simulink model "F16_mod"  (R2025b)
settings: Solver=ode4  StartTime=0  StopTime=Tend  FixedStep=0.01  RelTol=1e-3
values from neighbouring files (symbols this model uses):
  Param = load_F16_params()    [runF16_mod.m]
libraries: aerolibasang x3, aerolibobsolete x1, aerolibatmos2 x1
settings Model: Creator=sherpa  LastModifiedBy=karth
settings SolverCC: AlgebraicLoopSolver=TrustRegion
settings DataIOCC: SaveFormat=StructureWithTime
settings OptimizationCC: BlockReduction=off  DefaultParameterBehavior=Inlined  OptimizeBlockIOStorage=off  BufferReuse=off
settings DebuggingCC: AlgebraicLoopMsg=none  InitInArrayFormatMsg=none
settings ModelReferenceCC: EnableRefExpFcnMdlSchedulingChecks=on
settings RTWCC: GPUComputeCapability=3.5  DLArmComputeVersion=19.05

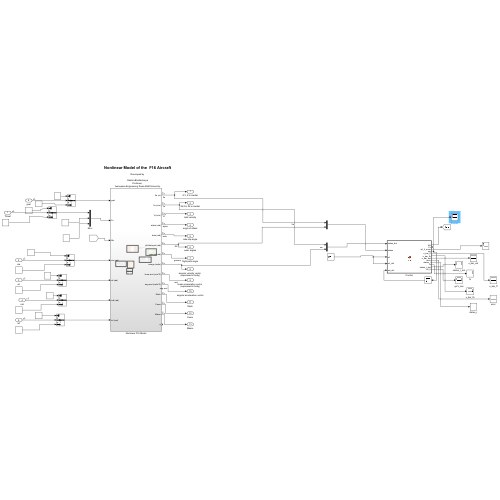
[thumbnail: Simulink's stored preview of the top-level diagram]
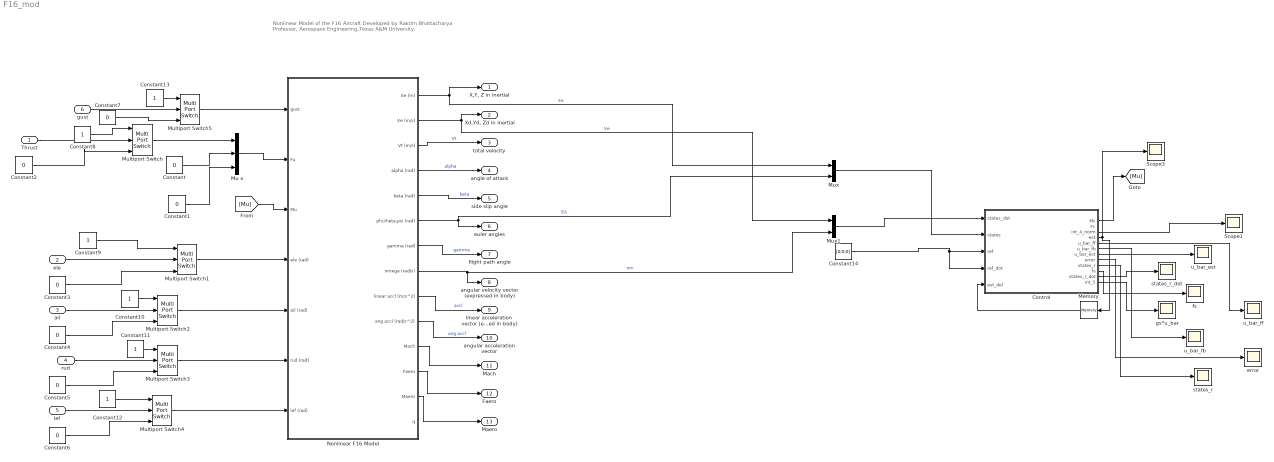
== system F16_mod ==
  note: Nonlinear Model of the F16 Aircraft
      |
      | Developed by
      |
      | Raktim Bhattacharya
      | Professor,
      | Aerospace Engineering,Texas A&M University.
  Thrust : Inport
  ele : Inport  Port=2
  ail : Inport  Port=3
  rud : Inport  Port=4
  lef : Inport  Port=5
  gust : Inport  Port=6
  Constant{,1..7} (8 alike) : Constant  Value=0
  Constant{8..13} (6 alike) : Constant
  Constant14 : Constant  Value=[0;0;0]
  Control : MATLAB Function  TreatAsAtomicUnit=on
  Memory : Memory  InitialCondition=[0;0;0]
  Mu x : Mux  Inputs=3
  Multiport Switch{,1..5} (6 alike) : MultiPortSwitch  DataPortOrder=Zero-based contiguous  Inputs=2  zeroidx=on  SaturateOnIntegerOverflow=off  InputSameDT=off
  Mux : Mux  Inputs=2
  Mux1 : Mux  Inputs=2
  Nonlinear F16 Model : Subsystem
  Scope1 : Scope
      settings: ActiveDisplayYMinimum=13407.32687  ActiveDisplayYMaximum=33407.32687  DataLoggingVariableName=ScopeData2
  Scope3 : Scope
      settings: ActiveDisplayYMinimum=-3.16857685066509  ActiveDisplayYMaximum=1.4182994151934736  DataLoggingVariableName=ScopeData4
  error : Scope
      settings: ActiveDisplayYMinimum=0.18819294431344591  ActiveDisplayYMaximum=1.6067438567419092  DataLoggingVariableName=ScopeData12
  fs : Scope
      settings: ActiveDisplayYMinimum=-3452.81147  ActiveDisplayYMaximum=2103.10858
  gs*u_bar : Scope
      settings: ActiveDisplayYMinimum=-2111.44761  ActiveDisplayYMaximum=3449.32295  DataLoggingVariableName=ScopeData2
  states_r : Scope
      settings: ActiveDisplayYMinimum=-1.0198079164284359  ActiveDisplayYMaximum=0.34149624108670595  DataLoggingVariableName=ScopeData3
  states_r_dot : Scope
      settings: ActiveDisplayYMinimum=-0.14936  ActiveDisplayYMaximum=0.22608  DataLoggingVariableName=ScopeData3
  u_bar_est : Scope
      settings: ActiveDisplayYMinimum=-0.14209  ActiveDisplayYMaximum=0.06478
  u_bar_fb : Scope
      settings: ActiveDisplayYMinimum=-1  ActiveDisplayYMaximum=1  DataLoggingVariableName=ScopeData11
  u_bar_ff : Scope
      settings: ActiveDisplayYMinimum=-3.90345245215E+6  ActiveDisplayYMaximum=3.513107206932E+7  DataLoggingVariableName=ScopeData15
  "X,Y, Z in inertial" : Outport
  "Xd,Yd, Zd in inertial" : Outport  Port=2
  total velocity : Outport  Port=3
  angle of attack : Outport  Port=4
  side slip angle : Outport  Port=5
  euler angles : Outport  Port=6
  flight path angle : Outport  Port=7
  angular velocity vector (expressed in body) : Outport  Port=8
  linear acceleration vector (expressed in body) : Outport  Port=9
  angular acceleration vector : Outport  Port=10
  Mach : Outport  Port=11
  Faero : Outport  Port=12
  Maero : Outport  Port=13
  wires:
  Nonlinear F16 Model/1(Xe (m)) -> "X,Y, Z in inertial"/1, Mux/1  "Xe"
  Nonlinear F16 Model/3(Vt (m/s)) -> total velocity/1  "Vt"
  Nonlinear F16 Model/4(alpha (rad)) -> angle of attack/1  "alpha"
  Nonlinear F16 Model/5(beta (rad)) -> side slip angle/1  "beta"
  Nonlinear F16 Model/7(gamma (rad)) -> flight path angle/1  "gamma"
  Nonlinear F16 Model/8(omega (rad/s)) -> angular velocity vector (expressed in body)/1, Mux1/2  "om"
  Nonlinear F16 Model/9(linear accl (m/s^2)) -> linear acceleration vector (expressed in body)/1  "accl"
  Nonlinear F16 Model/6(phi,theta,psi (rad)) -> euler angles/1, Mux/2  "EA"
  Nonlinear F16 Model/2(Ve (m/s)) -> "Xd,Yd, Zd in inertial"/1, Mux1/1  "Ve"
  Nonlinear F16 Model/10(ang accl (rad/s^2)) -> angular acceleration vector/1  "ang accl"
  Nonlinear F16 Model/11(Mach) -> Mach/1
  Nonlinear F16 Model/12(Faero) -> Faero/1
  Nonlinear F16 Model/13(Maero) -> Maero/1
  Control/1(Mc) -> [Mu]
  Control/5(u_bar_ff) -> u_bar_ff/1
  Control/9(states_r) -> states_r/1
  Control/6(u_bar_fb) -> u_bar_fb/1
  Control/3(int_4_norm) -> Scope1/1
  Memory/1 -> Control/5(est_del)
  Control/8(error) -> error/1
  Control/4(est) -> Memory/1, Scope3/1
  [Mu] -> Nonlinear F16 Model/3(Mu)
  Mux1/1 -> Control/1(states_dot)
  Constant/1 -> Mu x/2
  Mu x/1 -> Nonlinear F16 Model/2(Fu)
  Constant1/1 -> Mu x/3
  Thrust/1 -> Multiport Switch/2
  Multiport Switch/1 -> Mu x/1
  ele/1 -> Multiport Switch1/2
  Multiport Switch1/1 -> Nonlinear F16 Model/4(ele (rad))
  ail/1 -> Multiport Switch2/2
  Multiport Switch2/1 -> Nonlinear F16 Model/5(ail (rad))
  rud/1 -> Multiport Switch3/2
  Multiport Switch3/1 -> Nonlinear F16 Model/6(rud (rad))
  lef/1 -> Multiport Switch4/2
  Multiport Switch4/1 -> Nonlinear F16 Model/7(lef (rad))
  Constant2/1 -> Multiport Switch/3
  Constant3/1 -> Multiport Switch1/3
  Constant4/1 -> Multiport Switch2/3
  Constant5/1 -> Multiport Switch3/3
  Constant6/1 -> Multiport Switch4/3
  gust/1 -> Multiport Switch5/2
  Multiport Switch5/1 -> Nonlinear F16 Model/1(gust)
  Constant7/1 -> Multiport Switch5/3
  Constant8/1 -> Multiport Switch/1
  Constant9/1 -> Multiport Switch1/1
  Constant10/1 -> Multiport Switch2/1
  Constant11/1 -> Multiport Switch3/1
  Constant12/1 -> Multiport Switch4/1
  Constant13/1 -> Multiport Switch5/1
  Mux/1 -> Control/2(states)
  Constant14/1 -> Control/4(ref_dot), Control/3(ref)
  Control/7(u_bar_est) -> u_bar_est/1
  Control/10(fs) -> fs/1
  Control/12(int_5) -> gs*u_bar/1
  Control/11(states_r_dot) -> states_r_dot/1

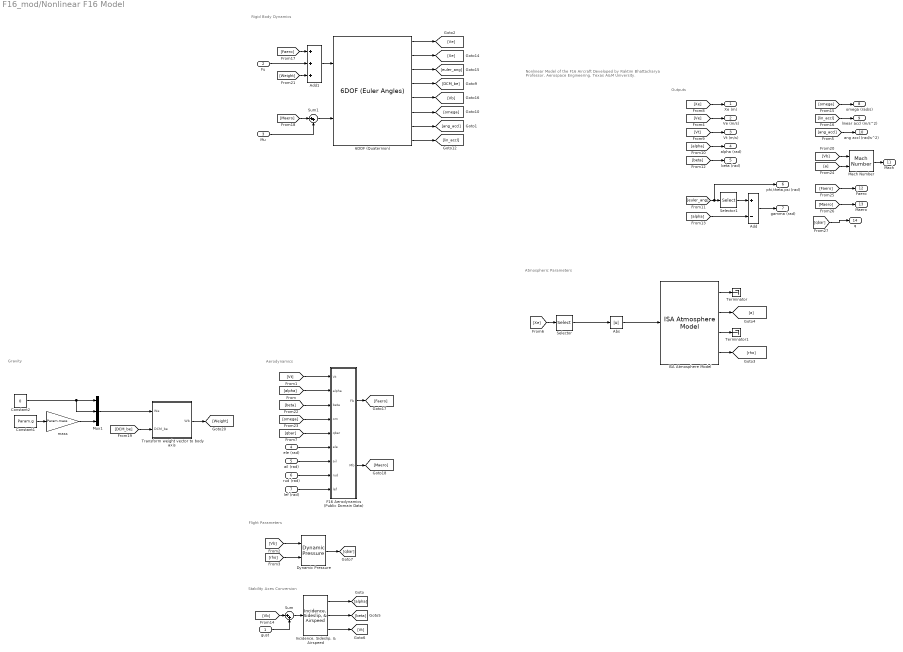
== system F16_mod/Nonlinear F16 Model ==
  note: Gravity
  note: Nonlinear Model of the F16 Aircraft
      |
      | Developed by Raktim Bhattacharya
      | Professor, Aerospace Engineering,
      | Texas A&M University.
  note: Aerodynamics
  note: Outputs
  note: Rigid Body Dynamics
  note: Stability Axes Conversion
  note: Atmospheric Parameters
  note: Flight Parameters
  gust : Inport  PortDimensions=3
  Fu : Inport  Port=2
  Mu : Inport  Port=3  PortDimensions=3
  ele (rad) : Inport  Port=4
  ail (rad) : Inport  Port=5
  rud (rad) : Inport  Port=6
  lef (rad) : Inport  Port=7
  6DOF (Quaternion) : aerolibobsolete/6DOF (Euler Angles)  units=Metric (MKS)  mtype=Fixed  rep=Euler Angles  xme_0=IC.inertial_position  Vm_0=IC.body_velocity  eul_0=IC.euler_angles  pm_0=IC.omega  mass_0=Param.mass  mass_e=0.5  mass_f=2.0  inertia=Param.moi  inertia_e=eye(3)  inertia_f=2*eye(3)  k_quat=1.0  vre_flag=on  abi_flag=off  aMode=0  xme_statename={'Xe', 'Ye', 'Ze'}  Vm_statename={'U', 'v', 'w'}  eul_statename=''  quat_statename={'qr', 'qi', 'qj', 'qk'}  pm_statename={'p', 'q', 'r'}  mass_statename=''
  Abs : Abs  SaturateOnIntegerOverflow=off
  Add : Sum  Inputs=+-
  Add1 : Sum  Inputs=+++
  Constant1 : Constant  Value=Param.g
  Constant2 : Constant  Value=0
  Dynamic Pressure : aerolibasang/Dynamic Pressure
  F16 Aerodynamics (Public Domain Data) : Subsystem
  ISA Atmosphere Model : aerolibatmos2/ISA Atmosphere Model  useExtended=off  action=Warning  custom=off  viscosityOut=off  g=9.80665  gamma=1.4  R=287.0531  L=0.0065  h_trop=11000  h_strat=20000  rho0=1.225  P0=101325  T0=288.15  h0=0  S=110.4  Tref=273.15  muref=1.716e-5
  "Incidence, Sideslip, & Airspeed" : aerolibasang/Incidence, Sideslip, & Airspeed
  Mach Number : aerolibasang/Mach Number
  Mux1 : Mux  Inputs=3
  Selector : Selector  InputPortWidth=3  IndexOptions=Index vector (dialog)  Indices=3  OutputSizes=1
  Selector1 : Selector  InputPortWidth=3  IndexOptions=Index vector (dialog)  Indices=2  OutputSizes=1
  Sum : Sum  Inputs=|++
  Sum1 : Sum  Inputs=|++
  Terminator : Terminator
  Terminator1 : Terminator
  Transform weight vector to body axis : MATLAB Function  TreatAsAtomicUnit=on
  mass : Gain  Gain=Param.mass
  Xe (m) : Outport
  Ve (m/s) : Outport  Port=2
  Vt (m/s) : Outport  Port=3
  alpha (rad) : Outport  Port=4
  beta (rad) : Outport  Port=5
  phi,theta,psi (rad) : Outport  Port=6
  gamma (rad) : Outport  Port=7
  omega (rad/s) : Outport  Port=8
  linear accl (m/s^2) : Outport  Port=9
  ang accl (rad/s^2) : Outport  Port=10
  Mach : Outport  Port=11
  Faero : Outport  Port=12
  Maero : Outport  Port=13
  q : Outport  Port=14
  wires:
  [Xe] -> Selector/1
  [beta] -> beta (rad)/1
  "Incidence, Sideslip, & Airspeed"/3 -> [Vt]
  ISA Atmosphere Model/3 -> Terminator1/1
  ISA Atmosphere Model/1 -> Terminator/1
  ISA Atmosphere Model/4 -> [rho]
  [rho] -> Dynamic Pressure/2
  [lin_accl] -> linear accl (m/s^2)/1
  [alpha] -> alpha (rad)/1
  ISA Atmosphere Model/2 -> [a]
  [Vb] -> Dynamic Pressure/1
  Add/1 -> gamma (rad)/1
  [Vt] -> Vt (m/s)/1
  "Incidence, Sideslip, & Airspeed"/2 -> [beta]
  Selector1/1 -> Add/1
  "Incidence, Sideslip, & Airspeed"/1 -> [alpha]
  Selector/1 -> Abs/1
  [alpha] -> Add/2
  [euler_ang] -> phi,theta,psi (rad)/1, Selector1/1
  [omega] -> omega (rad/s)/1
  Dynamic Pressure/1 -> [qbar]
  [Xe] -> Xe (m)/1
  Constant1/1 -> mass/1
  mass/1 -> Mux1/3
  Mux1/1 -> Transform weight vector to body axis/1(We)
  Transform weight vector to body axis/1(Wb) -> [Weight]
  [DCM_be] -> Transform weight vector to body axis/2(DCM_be)
  Constant2/1 -> Mux1/2, Mux1/1
  [Faero] -> Add1/1
  Fu/1 -> Add1/2
  [Weight] -> Add1/3
  Add1/1 -> 6DOF (Quaternion)/1
  [Vb] -> Sum/1
  Sum/1 -> "Incidence, Sideslip, & Airspeed"/1
  gust/1 -> Sum/2
  [Maero] -> Sum1/1
  Mu/1 -> Sum1/2
  6DOF (Quaternion)/1 -> [Ve]
  6DOF (Quaternion)/2 -> [Xe]
  6DOF (Quaternion)/3 -> [euler_ang]
  6DOF (Quaternion)/4 -> [DCM_be]
  6DOF (Quaternion)/5 -> [Vb]
  6DOF (Quaternion)/6 -> [omega]
  6DOF (Quaternion)/7 -> [ang_accl]
  6DOF (Quaternion)/8 -> [lin_accl]
  [Ve] -> Ve (m/s)/1
  [ang_accl] -> ang accl (rad/s^2)/1
  [Vb] -> Mach Number/1
  [a] -> Mach Number/2
  Mach Number/1 -> Mach/1
  F16 Aerodynamics (Public Domain Data)/1(Fb) -> [Faero]
  Sum1/1 -> 6DOF (Quaternion)/2
  F16 Aerodynamics (Public Domain Data)/2(Mb) -> [Maero]
  [Vt] -> F16 Aerodynamics (Public Domain Data)/1(Vt)
  [alpha] -> F16 Aerodynamics (Public Domain Data)/2(alpha)
  [beta] -> F16 Aerodynamics (Public Domain Data)/3(beta)
  [omega] -> F16 Aerodynamics (Public Domain Data)/4(om)
  [qbar] -> F16 Aerodynamics (Public Domain Data)/5(qbar)
  ele (rad)/1 -> F16 Aerodynamics (Public Domain Data)/6(ele)
  ail (rad)/1 -> F16 Aerodynamics (Public Domain Data)/7(ail)
  rud (rad)/1 -> F16 Aerodynamics (Public Domain Data)/8(rud)
  lef (rad)/1 -> F16 Aerodynamics (Public Domain Data)/9(lef)
  Abs/1 -> ISA Atmosphere Model/1
  [Faero] -> Faero/1
  [Maero] -> Maero/1
  [qbar] -> q/1

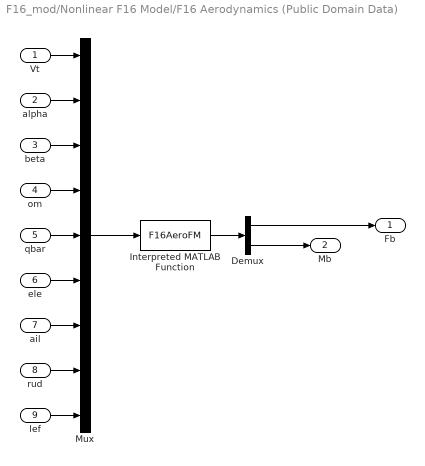
== system F16_mod/Nonlinear F16 Model/F16 Aerodynamics (Public Domain Data) ==
  Vt : Inport
  alpha : Inport  Port=2
  beta : Inport  Port=3
  om : Inport  Port=4
  qbar : Inport  Port=5
  ele : Inport  Port=6
  ail : Inport  Port=7
  rud : Inport  Port=8
  lef : Inport  Port=9
  Demux : Demux  Outputs=2
  Interpreted MATLAB Function : MATLABFcn  MATLABFcn=F16AeroFM  OutputDimensions=6
  Mux : Mux  Inputs=9
  Fb : Outport  PortDimensions=3
  Mb : Outport  Port=2  PortDimensions=3
  wires:
  om/1 -> Mux/4
  beta/1 -> Mux/3
  qbar/1 -> Mux/5
  alpha/1 -> Mux/2
  ele/1 -> Mux/6
  Vt/1 -> Mux/1
  ail/1 -> Mux/7
  rud/1 -> Mux/8
  lef/1 -> Mux/9
  Mux/1 -> Interpreted MATLAB Function/1
  Demux/1 -> Fb/1
  Demux/2 -> Mb/1
  Interpreted MATLAB Function/1 -> Demux/1

== matlab function F16_mod/Nonlinear F16 Model/Transform weight vector to body axis ==
  data: We input; Wb output; DCM_be input
function Wb = fcn(We,DCM_be)
Wb = DCM_be*We; % Weight in body coordinate system. DCM_be is correct, no need for transpose. They must have fixed it in this version.

== matlab function F16_mod/Control ==
  data: states_dot input; states input; Mc output; ref input; Fc output; int_4_norm output; ref_dot input; est output; est_del input; u_bar_ff output; u_bar_fb output; u_bar_est output; error output; states_r output; fs output; states_r_dot output; int_5 output
function [Mc,Fc,int_4_norm,est, u_bar_ff, u_bar_fb, u_bar_est,error, states_r, fs, states_r_dot, int_5]  = fcn(states_dot,states,ref,ref_dot,est_del)

states_r = states(4:6);
states_r_dot = states_dot(4:6);
ref_r = ref(1:3);
ref_r_dot = ref_dot(1:3);

error = states_r - ref_r;
error_dot = states_r_dot - ref_r_dot;

% theta = 0; % Placeholder angle (pitch) in radians
% phi = 

theta = states(5);
phi = states(4);

%% Aircraft Parameters from Simulator

slugs2kg = 14.5939;
ft2m     = 0.3048;

Param.S = 300*ft2m^2;      % Reference Area, m^2
Param.b =  30*ft2m;        % Wing Span, m
Param.cbar =  11.32*ft2m;     % Aerodynamic Mean Chord, m
Param.rho = 1.293;         % Air Density, kg/m^3
Param.xcgr = 0.35;         % reference center of gravity as a fraction of cbar
Param.xcg  = 0.30;         % center of gravity as a fraction of cbar.

%%%%%%%%%%%%%%% Testing With a Load %%%%%%%%%%%%%%%%%%%%%%%%%
%%%%%%%%%%%%%%% %%%%%%%%%%%%%%%%%%%%%%%%%%%%%%%%%%%%%%%%%%%%%


% % Asymmetric Parameters
% Param.S_asym = ;      % Reference Area, m^2
% Param.b_asym = ;        % Wing Span, m
% Param.cbar_asym = ;     % Aerodynamic Mean Chord, m
% Param.rho_asym = 1.293;         % Air Density, kg/m^3
% Param.xcgr_asym =;         % reference center of gravity as a fraction of cbar
% Param.xcg_asym  =;         % center of gravity as a fraction of cbar.



% Moment of Inertial
% Ixx = 9496.0;            % Principle Moment of Intertia around X-axis, slugs*ft^2
% Iyy = 55814.0;           % Principle Moment of Intertia around Y-axis, slugs*ft^2
% Izz = 63100.0;           % Principle Moment of Intertia around Z-axis, slugs*ft^2 
% Ixz = 982.0;           % Principle Moment of Intertia around XZ-axis,slugs*ft^2


% Moment of Inertial (With Load)
Ixx_w_load = 36698.21;            % Principle Moment of Intertia around X-axis, slugs*ft^2
Iyy_w_load =55826.33 ;           % Principle Moment of Intertia around Y-axis, slugs*ft^2
Izz_w_load = 63112.33;           % Principle Moment of Intertia around Z-axis, slugs*ft^2 
Ixz = 982.0;           % Principle Moment of Intertia around XZ-axis,slugs*ft^2

% Moment of Inertial (Asymmetric)
Ixx_asym = 229097.60 ;         % Principle Moment of Intertia around X-axis, slugs*ft^2
Iyy_asym = 55913.56 ;          % Principle Moment of Intertia around Y-axis, slugs*ft^2
Izz_asym = 63199.56;           % Principle Moment of Intertia around Z-axis, slugs*ft^2 
Ixz_asym = 982.0 ;             % Principle Moment of Intertia around XZ-axis,slugs*ft^2%
%Ixy_asym = 169.93;             % Principle Moment of Intertia around XY-axis,slugs*ft^2  -> KR 

% Moment of Inertial
Ixx = Ixx_asym;            % Principle Moment of Intertia around X-axis, slugs*ft^2
Iyy = Iyy_asym;           % Principle Moment of Intertia around Y-axis, slugs*ft^2
Izz = Izz_asym;           % Principle Moment of Intertia around Z-axis, slugs*ft^2 
Ixz = Ixz;           % Principle Moment of Intertia around XZ-axis,slugs*ft^2
Param.moi_asym = [Ixx 0 Ixz;
            0   Iyy 0
            Ixz 0   Izz]*slugs2kg*(ft2m)^2; % Convert to Kg*m^2
I_asym = [Ixx 0 Ixz;
            0   Iyy 0
            Ixz 0   Izz]*slugs2kg*(ft2m)^2; % Convert to Kg*m^2


%Param.mass = 636.94*slugs2kg;     % kg%

Param.mass_asym =12295 ;     % kg
Param.g = 9.806;  % m/s^2

%%


m_aircraft = Param.mass_asym;
%l_aircraft = 15.06;
%wingspan = Param.b;
%wing_area = Param.S;
%wing_width = 9.96;
m_load = 1000; 
%r_load = 0.3;
n = 4;
%wing_mass = 0.12 * m_aircraft;  % this is the combined mass of both wings
%r_fuselage = 1.5;
%wingspan_new = wingspan - r_fuselage *  2;
m_sym = m_aircraft + n * m_load;
%m_asym = m_aircraft + (n-1) * m_load;
%m_aircraft_prime = m_aircraft - m_load; % KR

%I_fuselage_origin = 0.5 * (m_aircraft - wing_mass) * r_fuselage.^2;
%I_wings = 2 * (1/12) * (wing_mass) * (2 * wing_width.^2);
%I_load = n * ((0.5 * m_load * r_load.^2) + (m_load * wing_width.^2));
%I_sym = I_fuselage_origin + I_wings + I_load;
%cg_x_sym = 0;
%cg_y_sym = 0;
%cg_z_sym = 0;
%cg_shift = (m_aircraft * 0 + (n/2)*m_load - (n/2-1)*m_load)/m_asym; % = 0.0813
g = Param.g;

%I_asym = diag([1.5e4, 2.0e4, 2.5e4]); % Diagonal terms (kg·m²)
%I_xx_asym = 1.5e4; 
%I_yy_asym = 2.0e4;
%I_zz_asym = 2.5e4;

%I_xz_asym = 0.02 * I_xx_asym; % Small cross-term (2% of I_xx)
%I_yz_asym = 0.02 * I_yy_asym; 
%I_xy_asym = 0.02 * I_zz_asym; 
I_xx_sym = Ixx*slugs2kg*(ft2m)^2;
I_yy_sym = Iyy*slugs2kg*(ft2m)^2;
I_zz_sym = Izz*slugs2kg*(ft2m)^2;
I_xz_sym = Ixz*slugs2kg*(ft2m)^2;
I_xy_sym = 0*slugs2kg*(ft2m)^2;
I_yz_sym = 0*slugs2kg*(ft2m)^2;

I_sym = [I_xx_sym I_xy_sym I_xz_sym;
         I_xy_sym I_yy_sym I_yz_sym;
         I_xz_sym I_yz_sym I_zz_sym];

I_master = I_asym;

%I_prime = 0; %KR

Zcm = 0; 
Ycm = 0;
Xcm = Param.xcg*Param.cbar;

%%

Fx = 0;
Fy = 0;
Fz = 0;
Fs = [Fx;
     Fy;
     Fz];

Ms = [0;0;0];
Mxs = Ms(1);
Mys = Ms(2);
Mzs = Ms(3);

p = states_dot(1);
q = states_dot(2);
r = states_dot(3);
u = states_dot(4);
v = states_dot(5);
w = states_dot(6);

% M = [
%     1 0 0 0 Zcm -Ycm; 
%     0 1 0 -Zcm 0 Xcm; 
%     0 0 1 Ycm -Xcm 0; 
%     0 -m_asym*Zcm m_asym*Ycm I_xx_asym -I_xy_asym -I_xz_asym; 
%     m_asym*Zcm 0 -m_asym*Xcm -I_xy_asym I_yy_asym -I_yz_asym; 
%     -m_asym*Ycm m_asym*Xcm 0 -I_xz_asym -I_yz_asym I_zz_asym
%     ];

% S_dot = [
%     u_dot; 
%     v_dot; 
%     w_dot; 
%     p_dot; 
%     q_dot; 
%     r_dot
%     ];

% C = [
%     -q*w + r*v + (q.^2 + r.^2)*Xcm - p*q*Ycm - r*p*Zcm;
%     -r*u + p*w + (r.^2 + p.^2)*Ycm - p*q*Xcm - q*r*Zcm;
%     -p*v + q*u + (p.^2 + q.^2)*Zcm - r*p*Xcm - q*r*Ycm;
%     I_xz_asym*p*q + (I_yy_asym-I_zz_asym)*q*r - I_xy_asym*r*p + I_yz_asym*(q.^2-r.^2) + m_sym*(q*u - p*v)*Ycm + m_sym*(r*u-p*w)*Zcm;
%     (-I_yz_asym)*p*q + I_xy_asym*q*r - (I_zz_asym-I_xx_asym)*r*p + I_xz_asym*(r.^2-p.^2) + m_sym*(p*v - q*u)*Xcm + m_sym*(r*v-q*w)*Zcm;
%     (I_xx_asym-I_yy_asym)*p*q - I_xz_asym*q*r - I_yz_asym*r*p + I_xy_asym*(p.^2-q.^2) + m_sym*(p*w - r*u)*Xcm + m_sym*(q*w-r*v)*Ycm
%     ];

% A = [
%     -g*sin(theta);
%     g*cos(theta)*sin(phi);
%     g*cos(theta)*cos(phi);
%     (-Zcm)*m_sym*g*cos(theta)*sin(phi) + Ycm*m_sym*g*cos(theta)*cos(phi);
%     (-Zcm)*m_sym*g*sin(theta) - Xcm*m_sym*g*cos(theta)*cos(phi);
%     Ycm*m_sym*g*sin(theta) + Xcm*m_sym*g*cos(theta)*sin(phi)
%     ];

A = [0 -m_sym*Zcm m_sym*Ycm; m_sym*Zcm 0 -m_sym*Xcm; -m_sym*Ycm m_sym*Xcm 0];

% D = [
%     (1/m_sym) 0 0 0 0 0;
%     0 (1/m_sym) 0 0 0 0;
%     0 0 (1/m_sym) 0 0 0;
%     0 0 0 1 0 0;
%     0 0 0 0 1 0;
%     0 0 0 0 0 1
%     ];

% U = [
%     Fx;
%     Fy;
%     Fz;
%     Mx;
%     My;
%     Mz
%     ];

% S_dot = inv(M) * (C + A) + inv(M) * D * U;

%F1_t = -q*w + r*v + (q.^2 + r.^2)*Xcm - p*q*Ycm - r*p*Zcm + (1/m_asym)*Fx;
%F2_t = -r*u + p*w + (r.^2 + p.^2)*Ycm - p*q*Xcm - q*r*Zcm + (1/m_asym)*Fy;
%F3_t = -p*v + q*u + (p.^2 + q.^2)*Zcm - r*p*Xcm - q*r*Ycm + (1/m_asym)*Fz;
%F = [F1_t;F2_t;F3_t];


F1_t = -q*w + r*v + (q.^2 + r.^2)*Xcm - p*q*Ycm - r*p*Zcm + (1/m_sym)*Fx;
F2_t = -r*u + p*w + (r.^2 + p.^2)*Ycm - p*q*Xcm - q*r*Zcm + (1/m_sym)*Fy;
F3_t = -p*v + q*u + (p.^2 + q.^2)*Zcm - r*p*Xcm - q*r*Ycm + (1/m_sym)*Fz;
F=[F1_t;F2_t;F3_t];

%M1_t = I_xz_asym*p*q + (I_yy_asym-I_zz_asym)*q*r - I_xy_asym*r*p + I_yz_asym*(q.^2-r.^2) + m_asym*(q*u - p*v)*Ycm + m_asym*(r*u-p*w)*Zcm + (-Zcm)*m_asym*g*cos(theta)*sin(phi) + Ycm*m_asym*g*cos(theta)*cos(phi);
%M2_t = (-I_yz_asym)*p*q + I_xy_asym*q*r - (I_zz_asym-I_xx_asym)*r*p + I_xz_asym*(r.^2-p.^2) + m_asym*(p*v - q*u)*Xcm + m_asym*(r*v-q*w)*Zcm + (-Zcm)*m_asym*g*sin(theta) - Xcm*m_asym*g*cos(theta)*cos(phi);
%M3_t = (I_xx_asym-I_yy_asym)*p*q - I_xz_asym*q*r - I_yz_asym*r*p + I_xy_asym*(p.^2-q.^2) + m_asym*(p*w - r*u)*Xcm + m_asym*(q*w-r*v)*Ycm + Ycm*m_asym*g*sin(theta) + Xcm*m_asym*g*cos(theta)*sin(phi);
%Mi = [M1_t; M2_t; M3_t];

% M1_t = I_xz_asym*p*q + (I_yy_asym-I_zz_asym)*q*r - I_xy_asym*r*p + I_yz_asym*(q.^2-r.^2) + m_asym*(q*u - p*v)*Ycm + m_asym*(r*u-p*w)*Zcm + (-Zcm)*m_asym*g*cos(theta)*sin(phi) + Ycm*m_asym*g*cos(theta)*cos(phi);
% M2_t = (-I_yz_asym)*p*q + I_xy_asym*q*r + (I_zz_asym-I_xx_asym)*r*p + I_xz_asym*(r.^2-p.^2) + m_asym*(p*v - q*u)*Xcm + m_asym*(r*v-q*w)*Zcm + (-Zcm)*m_asym*g*sin(theta) - Xcm*m_asym*g*cos(theta)*cos(phi);
% M3_t = (I_xx_asym-I_yy_asym)*p*q - I_xz_asym*q*r - I_yz_asym*r*p + I_xy_asym*(p.^2-q.^2) + m_asym*(p*w - r*u)*Xcm + m_asym*(q*w-r*v)*Ycm + Ycm*m_asym*g*sin(theta) + Xcm*m_asym*g*cos(theta)*sin(phi);
% Mi = [M1_t; M2_t; M3_t];

% M1_t = I_xz_sym*p*q + (I_yy_sym-I_zz_sym)*q*r - I_xy_sym*r*p + I_yz_sym*(q.^2-r.^2) + m_sym*(q*u - p*v)*Ycm + m_sym*(r*u-p*w)*Zcm + (-Zcm)*m_sym*g*cos(theta)*sin(phi) + Ycm*m_sym*g*cos(theta)*cos(phi);
% M2_t = (-I_yz_sym)*p*q + I_xy_sym*q*r + (I_zz_sym-I_xx_sym)*r*p + I_xz_sym*(r.^2-p.^2) + m_sym*(p*v - q*u)*Xcm + m_sym*(r*v-q*w)*Zcm + (-Zcm)*m_sym*g*sin(theta) - Xcm*m_sym*g*cos(theta)*cos(phi);
% M3_t = (I_xx_sym-I_yy_sym)*p*q - I_xz_sym*q*r - I_yz_sym*r*p + I_xy_sym*(p.^2-q.^2) + m_sym*(p*w - r*u)*Xcm + m_sym*(q*w-r*v)*Ycm + Ycm*m_sym*g*sin(theta) + Xcm*m_sym*g*cos(theta)*sin(phi);
% Mi = [M1_t; M2_t; M3_t];

M1_t = I_xz_sym*p*q + (I_yy_sym-I_zz_sym)*q*r - I_xy_sym*r*p + I_yz_sym*(q.^2-r.^2) + m_sym*(q*u - p*v)*Ycm + m_sym*(r*u-p*w)*Zcm + (-Zcm)*m_sym*g*cos(theta)*sin(phi) + Ycm*m_sym*g*cos(theta)*cos(phi);
M2_t = (-I_yz_sym)*p*q + I_xy_sym*q*r + (I_zz_sym-I_xx_sym)*r*p + I_xz_sym*(r.^2-p.^2) + m_sym*(p*v - q*u)*Xcm + m_sym*(r*v-q*w)*Zcm + (-Zcm)*m_sym*g*sin(theta) - Xcm*m_sym*g*cos(theta)*cos(phi);
M3_t = (I_xx_sym-I_yy_sym)*p*q - I_xz_sym*q*r - I_yz_sym*r*p + I_xy_sym*(p.^2-q.^2) + m_sym*(p*w - r*u)*Xcm + m_sym*(q*w-r*v)*Ycm + Ycm*m_sym*g*sin(theta) + Xcm*m_sym*g*cos(theta)*sin(phi);
Mi = [M1_t; M2_t; M3_t];

int_1 = -A*(F);          % KR
int_2 = -A*(Fs)/m_sym; % KR
int_3 = Mi + Ms; % KR
int_4 = ((1/m_sym)*(A^2)) + I_master; % KR

fs = inv(int_4) * (int_1 + int_2 + int_3); %KR

gs = (((A^2/m_sym) + I_master)); %KR Does Myc and Mzc also have to be included in the function definition above?

int_4_norm = norm(int_4,2);
gs_norm = norm(gs,2);

K = diag([5;5;5]);

u_bar_ff = -inv(gs)*(fs);

u_bar_est = inv(gs)*(est_del);

u_bar_fb = -inv(gs)*(K*error);

u_bar = u_bar_ff + u_bar_est + u_bar_fb;  %ffffffhgb

Fc = [0;0;0];
Mc = u_bar;
int_5 = gs*(u_bar);

est = states_r_dot - fs - ((gs)*u_bar);
